simulink model "vloopControl"  (R2023b)
settings: Solver=ode15s  StartTime=0.0  StopTime=1.0  RelTol=1e-3  EnableMultiTasking=on
InitFcn:
  | G = 107.815;
libraries: simulink x1, roblocks x1
Description:
  | vloop parameters for
  | Puma560 shoulder joint
  | with link inertia
  | RVC1 p.205
settings Model: DisableUpgradeWarningsForVersion=R2014b  Creator=pic  LastModifiedBy=dell
settings SolverCC: AlgebraicLoopSolver=TrustRegion
settings DataIOCC: LimitDataPoints=on  SaveFormat=Array  SignalLoggingSaveFormat=ModelDataLogs  TimeSaveName=t  OutputSaveName=y
settings OptimizationCC: ExpressionDepthLimit=2147483647  LifeSpan=inf
settings DebuggingCC: UnderspecifiedInitializationDetection=Classic  MergeDetectMultiDrivingBlocksExec=none  SolverPrmCheckMsg=warning  MultiTaskRateTransMsg=warning  FcnCallInpInsideContextMsg=warning  UnconnectedInputMsg=warning  UnconnectedOutputMsg=warning  UnconnectedLineMsg=warning  AllowSymbolicDim=off  StateNameClashWarn=warning  SFUnexpectedBacktrackingDiag=warning  SFNoUnconditionalDefaultTransitionDiag=warning  SFExecutionAtInitializationDiag=none  ArithmeticOperatorsInVariantConditions=warning
settings HardwareCC: ProdBitPerPointer=32  ProdBitPerSizeT=32  ProdBitPerPtrDiffT=32  ProdLargestAtomicFloat=None  ProdIntDivRoundTo=Undefined  ProdEndianess=Unspecified  ProdWordSize=32  ProdHWDeviceType=32-bit Generic
settings ModelReferenceCC: EnableRefExpFcnMdlSchedulingChecks=on  PropagateSignalLabelsOutOfModel=off
settings SFSimCC: SimUseLocalCustomCode=off  CustomCodeUndefinedFunction=UseInterfaceOnly
settings SFSimCC: SimCustomInitializer=|
  | if ~exist(tau_d)
  |    tau_d = 0
  | end
settings RTWCC: RTWUseLocalCustomCode=off
settings CodeAppCC: StateflowObjectComments=on
settings GRTTargetCC: TargetLangStandard=C89/C90 (ANSI)  CombineOutputUpdateFcns=off  GRTInterface=on
settings ConfigComp: CovMetricSettings=dw  CovSaveCumulativeToWorkspaceVar=on  CovSaveSingleToWorkspaceVar=on  CovExternalEMLEnable=off  CovSFcnEnable=off

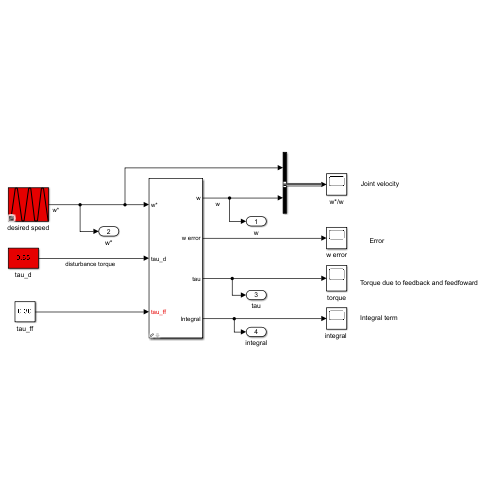
[thumbnail: Simulink's stored preview of the top-level diagram]
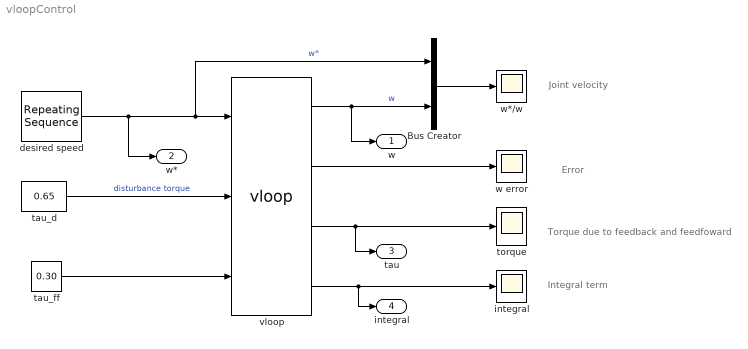
== system vloopControl ==
  note: Integral term
  note: Torque due to feedback and feedfoward
  note: Error
  note: Joint velocity
  Bus Creator : BusCreator  Inputs=2
  desired speed : simulink/Sources/Repeating Sequence  rep_seq_t=[0 1 3 4 6]/10  rep_seq_y=[0 0 50 50 0]
  "integral " : Scope
  tau_d : Constant  Value=0.65
  tau_ff : Constant  Value=0.30
  torque : Scope
  vloop : roblocks/Arm/vloop  J=580e-6  B=817e-6  Km=0.228  tau_max=0.9  Kv=1  Ki=10  T=0.001
  w error : Scope
  w*/w : Scope
  w : Outport
  w* : Outport  Port=2
  tau : Outport  Port=3
  integral : Outport  Port=4
  wires:
  desired speed/1 -> w*/1, Bus Creator/1, vloop/1  "w*"
  Bus Creator/1 -> w*/w/1
  vloop/1 -> Bus Creator/2, w/1  "w"
  vloop/2 -> w error/1
  vloop/3 -> tau/1, torque/1
  vloop/4 -> integral/1, "integral "/1
  tau_d/1 -> vloop/2  "disturbance torque"
  tau_ff/1 -> vloop/3
